simulink model "ROS_plant"  (R2020a)
settings: Solver=VariableStepAuto  StartTime=0.0  StopTime=30  MaxStep=1e-03
values from neighbouring files (symbols this model uses):
  g = 9.81    [StateFeedbackControl2.m]
  jx = 0.0196    [StateFeedbackControl2.m]
  jy = 0.0196    [StateFeedbackControl2.m]
  jz = 0.0264    [StateFeedbackControl2.m]
  m = 0.5    [StateFeedbackControl2.m]
  xo = [P_star; zeros(9,1)]    [StateFeedbackControl2.m]
undefined symbols (not defined in the file or in its folder): Pose, Twist, X, Y, Z
libraries: robotlib x5
settings Model: Creator=carlopellettieri  LastModifiedBy=carlopellettieri

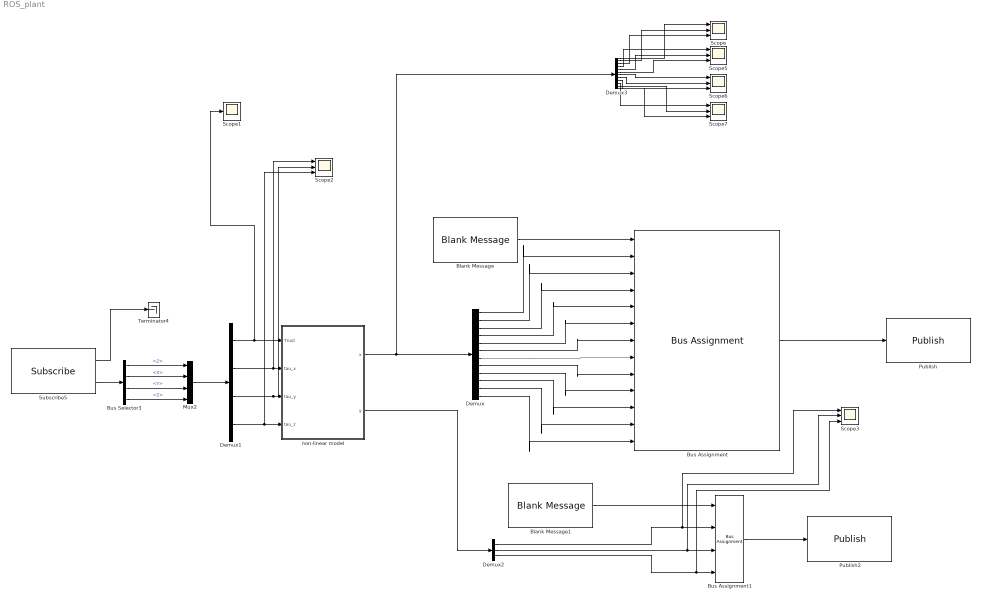
== system ROS_plant ==
  Blank Message : robotlib/Blank Message  messageClass=Message  entityType=nav_msgs/Odometry  messageType=nav_msgs/Odometry  SampleTime=inf
  Blank Message1 : robotlib/Blank Message  messageClass=Message  entityType=geometry_msgs/Point  messageType=geometry_msgs/Point  SampleTime=inf
  Bus Assignment : BusAssignment  AssignedSignals=Pose.Pose.Position.X,Pose.Pose.Position.Y,Pose.Pose.Position.Z,Twist.Twist.Linear.X,Twist.Twist.Linear.Y,Twist.Twist.Linear.Z,Pose.Pose.Orientation.X,Pose.Pose.Orientation.Y,Pose.Pose.Orientation.Z,Twist.Twist.Angular.X,Twist.Twist.Angular.Y,Twist.Twist.Angular.Z
  Bus Assignment1 : BusAssignment  AssignedSignals=X,Y,Z
  Bus Selector3 : BusSelector  OutputSignals=Force.Z,Torque.X,Torque.Y,Torque.Z
  Demux : Demux  Outputs=12
  Demux1 : Demux
  Demux2 : Demux  Outputs=3
  Demux3 : Demux  Outputs=12
  Mux2 : Mux
  Publish : robotlib/Publish  topicSource=Select from ROS network  topic=/x  messageType=nav_msgs/Odometry  messageQueueLength=1
  Publish2 : robotlib/Publish  topicSource=Select from ROS network  topic=/y_out  messageType=geometry_msgs/Point  messageQueueLength=1
  Scope{,2..3,5..7} (6 alike) : Scope  NumInputPorts=3
  Scope1 : Scope
  Subscribe5 : robotlib/Subscribe  topicSource=Select from ROS network  topic=/u  messageType=geometry_msgs/Wrench  sampleTime=-1  messageQueueLength=1
  Terminator4 : Terminator
  non-linear model : Subsystem
  wires:
  Demux/3 -> Bus Assignment/4
  Demux1/4 -> non-linear model/4(tau_z), Scope2/3
  Blank Message1/1 -> Bus Assignment1/1
  Demux/7 -> Bus Assignment/8
  Demux/4 -> Bus Assignment/5
  Demux/2 -> Bus Assignment/3
  Bus Selector3/2 -> Mux2/2  "<X>"
  Demux/5 -> Bus Assignment/6
  Bus Selector3/4 -> Mux2/4  "<Z>"
  Demux/10 -> Bus Assignment/11
  Demux/1 -> Bus Assignment/2
  Demux1/1 -> Scope1/1, non-linear model/1(Trust)
  Demux1/3 -> Scope2/2, non-linear model/3(tau_y)
  Blank Message/1 -> Bus Assignment/1
  Subscribe5/1 -> Terminator4/1
  Bus Assignment1/1 -> Publish2/1
  Demux/12 -> Bus Assignment/13
  Mux2/1 -> Demux1/1
  Bus Selector3/3 -> Mux2/3  "<Y>"
  Demux/9 -> Bus Assignment/10
  Demux2/3 -> Scope3/3, Bus Assignment1/4
  Demux/11 -> Bus Assignment/12
  Subscribe5/2 -> Bus Selector3/1
  non-linear model/2(y) -> Demux2/1
  Demux/8 -> Bus Assignment/9
  non-linear model/1(x) -> Demux3/1, Demux/1
  Bus Selector3/1 -> Mux2/1  "<Z>"
  Bus Assignment/1 -> Publish/1
  Demux/6 -> Bus Assignment/7
  Demux1/2 -> Scope2/1, non-linear model/2(tau_x)
  Demux2/1 -> Scope3/1, Bus Assignment1/2
  Demux2/2 -> Scope3/2, Bus Assignment1/3
  Demux3/1 -> Scope/1
  Demux3/2 -> Scope/2
  Demux3/3 -> Scope/3
  Demux3/4 -> Scope5/1
  Demux3/5 -> Scope5/2
  Demux3/6 -> Scope5/3
  Demux3/7 -> Scope6/1
  Demux3/8 -> Scope6/2
  Demux3/9 -> Scope6/3
  Demux3/10 -> Scope7/1
  Demux3/11 -> Scope7/2
  Demux3/12 -> Scope7/3

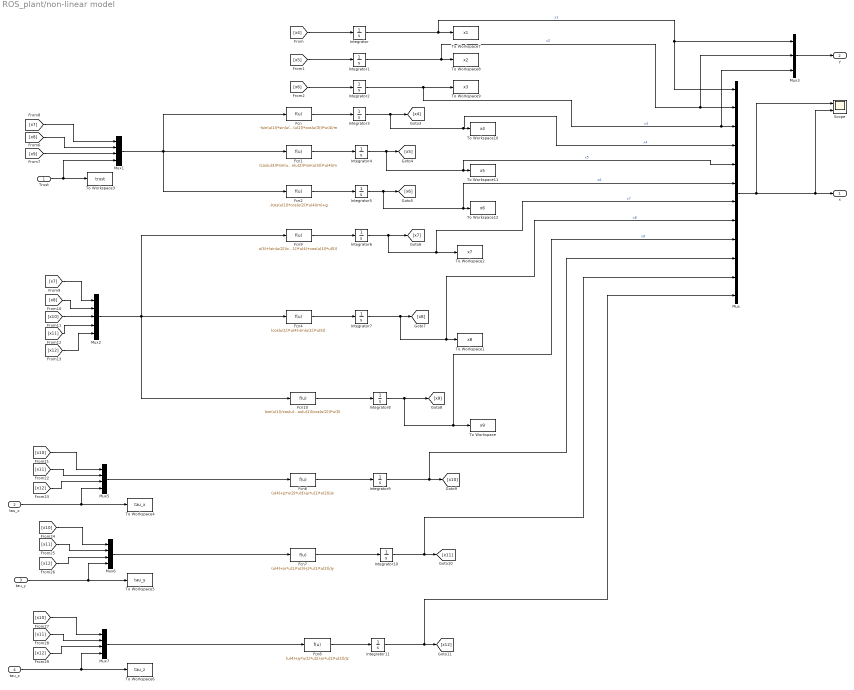
== system ROS_plant/non-linear model ==
  Trust : Inport
  tau_x : Inport  Port=2
  tau_y : Inport  Port=3
  tau_z : Inport  Port=4
  Fcn : Fcn  Expr=-(sin(u(1))*sin(u(3))+cos(u(1))*sin(u(2))*cos(u(3)))*u(4)/m
  Fcn1 : Fcn  Expr=(cos(u(3))*sin(u(1))-cos(u(1))*sin(u(2))*sin(u(3)))*u(4)/m
  Fcn10 : Fcn  Expr=(sin(u(1))/cos(u(2)))*u(4)+(cos(u(1))/cos(u(2)))*u(5)
  Fcn2 : Fcn  Expr=-(cos(u(1))*cos(u(2))*u(4)/m)+g
  Fcn4 : Fcn  Expr=(cos(u(1))*u(4)-sin(u(1))*u(5))
  Fcn6 : Fcn  Expr=(u(4)+jz*u(2)*u(3)-jy*u(1)*u(2))/jx
  Fcn7 : Fcn  Expr=(u(4)+jx*u(1)*u(3)-jz*u(1)*u(2))/jy
  Fcn8 : Fcn  Expr=(u(4)+jy*u(1)*u(2)-jx*u(1)*u(2))/jz
  Fcn9 : Fcn  Expr=u(3)+(sin(u(2))/cos(u(2)))*(sin(u(1))*u(4)+cos(u(1))*u(5))
  Integrator : Integrator  InitialCondition=xo(1)
  Integrator1 : Integrator  InitialCondition=xo(2)
  Integrator10 : Integrator  InitialCondition=xo(11)
  Integrator11 : Integrator  InitialCondition=xo(12)
  Integrator2 : Integrator  InitialCondition=xo(3)
  Integrator3 : Integrator  InitialCondition=xo(4)
  Integrator4 : Integrator  InitialCondition=xo(5)
  Integrator5 : Integrator  InitialCondition=xo(6)
  Integrator6 : Integrator  InitialCondition=xo(7)
  Integrator7 : Integrator  InitialCondition=xo(8)
  Integrator8 : Integrator  InitialCondition=xo(9)
  Integrator9 : Integrator  InitialCondition=xo(10)
  Mux : Mux  Inputs=12
  Mux{1,5..7} (4 alike) : Mux
  Mux2 : Mux  Inputs=5
  Mux3 : Mux  Inputs=3
  Scope : Scope  NumInputPorts=2
  To Workspace : ToWorkspace  VariableName=x9  SaveFormat=Timeseries  SampleTime=-1
  To Workspace1 : ToWorkspace  VariableName=x8  SaveFormat=Timeseries  SampleTime=-1
  To Workspace10 : ToWorkspace  VariableName=x4  SaveFormat=Timeseries  SampleTime=-1
  To Workspace11 : ToWorkspace  VariableName=x5  SaveFormat=Timeseries  SampleTime=-1
  To Workspace12 : ToWorkspace  VariableName=x6  SaveFormat=Timeseries  SampleTime=-1
  To Workspace2 : ToWorkspace  VariableName=x7  SaveFormat=Timeseries  SampleTime=-1
  To Workspace3 : ToWorkspace  VariableName=trust  SaveFormat=Timeseries  SampleTime=-1
  To Workspace4 : ToWorkspace  VariableName=tau_x  SaveFormat=Timeseries  SampleTime=-1
  To Workspace5 : ToWorkspace  VariableName=tau_y  SaveFormat=Timeseries  SampleTime=-1
  To Workspace6 : ToWorkspace  VariableName=tau_z  SaveFormat=Timeseries  SampleTime=-1
  To Workspace7 : ToWorkspace  VariableName=x1  SaveFormat=Timeseries  SampleTime=-1
  To Workspace8 : ToWorkspace  VariableName=x2  SaveFormat=Timeseries  SampleTime=-1
  To Workspace9 : ToWorkspace  VariableName=x3  SaveFormat=Timeseries  SampleTime=-1
  x : Outport
  y : Outport  Port=2
  wires:
  Integrator5/1 -> Mux/6, To Workspace12/1, [x6]  "x6"
  Fcn9/1 -> Integrator6/1
  Integrator6/1 -> Mux/7, To Workspace2/1, [x7]  "x7"
  Integrator3/1 -> Mux/4, To Workspace10/1, [x4]  "x4"
  Integrator/1 -> Mux/1, Mux3/1, To Workspace7/1  "x1"
  Fcn2/1 -> Integrator5/1
  Integrator4/1 -> Mux/5, To Workspace11/1, [x5]  "x5"
  Integrator1/1 -> Mux3/2, Mux/2, To Workspace8/1  "x2"
  Integrator2/1 -> Mux3/3, Mux/3, To Workspace9/1  "x3"
  Fcn1/1 -> Integrator4/1
  Integrator7/1 -> Mux/8, To Workspace1/1, [x8]  "x8"
  Fcn4/1 -> Integrator7/1
  Fcn10/1 -> Integrator8/1
  Integrator8/1 -> Mux/9, To Workspace/1, [x9]  "x9"
  Integrator11/1 -> Mux/12, [x12]
  Integrator9/1 -> Mux/10, [x10]
  Integrator10/1 -> Mux/11, [x11]
  Fcn/1 -> Integrator3/1
  [x4] -> Integrator/1
  [x6] -> Integrator2/1
  [x5] -> Integrator1/1
  Mux1/1 -> Fcn2/1, Fcn1/1, Fcn/1
  Mux2/1 -> Fcn9/1, Fcn4/1, Fcn10/1
  Fcn6/1 -> Integrator9/1
  Mux5/1 -> Fcn6/1
  Mux6/1 -> Fcn7/1
  Fcn7/1 -> Integrator10/1
  Mux7/1 -> Fcn8/1
  Fcn8/1 -> Integrator11/1
  [x8] -> Mux1/2
  Trust/1 -> To Workspace3/1, Mux1/4
  [x7] -> Mux1/1
  [x9] -> Mux1/3
  [x10] -> Mux2/3
  [x12] -> Mux2/5
  [x7] -> Mux2/1
  [x11] -> Mux2/4
  [x8] -> Mux2/2
  tau_x/1 -> Mux5/4, To Workspace4/1
  [x11] -> Mux5/2
  [x10] -> Mux5/1
  [x12] -> Mux5/3
  [x10] -> Mux6/1
  [x11] -> Mux6/2
  [x12] -> Mux6/3
  tau_y/1 -> Mux6/4, To Workspace5/1
  [x10] -> Mux7/1
  [x11] -> Mux7/2
  [x12] -> Mux7/3
  tau_z/1 -> Mux7/4, To Workspace6/1
  Mux/1 -> Scope/2, x/1, Scope/1
  Mux3/1 -> y/1
